simulink model "canudas_goal2"  (R2012b)
settings: Solver=FixedStepDiscrete  StartTime=0.0  StopTime=Inf  FixedStep=0.033  RelTol=1e-3
values from neighbouring files (symbols this model uses):
  eps1 = 0.005    [param.m]
  eps2 = 1*2*pi/360    (= 0.0174532925199)    [param.m]
  k1 = 1.35/4    (= 0.3375)    [param.m]
  k2 = 4.6/4    (= 1.15)    [param.m]
  max_phi = 48000*6.9440e-06/r    (= 16.2591219512)    [param.m]
  max_v = r * max_phi    (= 0.333312)    [param.m]
  max_w = max_phi*2*r/l    (= 7.54014251781)    [param.m]
  thetar = pi    (= 3.14159265359)    [param.m]
  xr = 0    [param.m]
  yr = 0    [param.m]
libraries: simiam x5, simulink x1, simulink_extras x1
settings Model: Creator=jdelacroix  LastModifiedBy=samati
settings DataIOCC: SignalLoggingSaveFormat=ModelDataLogs  SaveOutput=off  SaveTime=off
settings DebuggingCC: MultiTaskDSMMsg=warning  MultiTaskCondExecSysMsg=none  FcnCallInpInsideContextMsg=EnableAllAsWarning  StrictBusMsg=None
settings RTWCC: IncludeERTFirstTime=on
settings CodeAppCC: CustomSymbolStrType=$N$R$M_T  InternalIdentifier=Shortened
settings GRTTargetCC: CodeReplacementLibrary=None  CPPClassGenCompliant=on

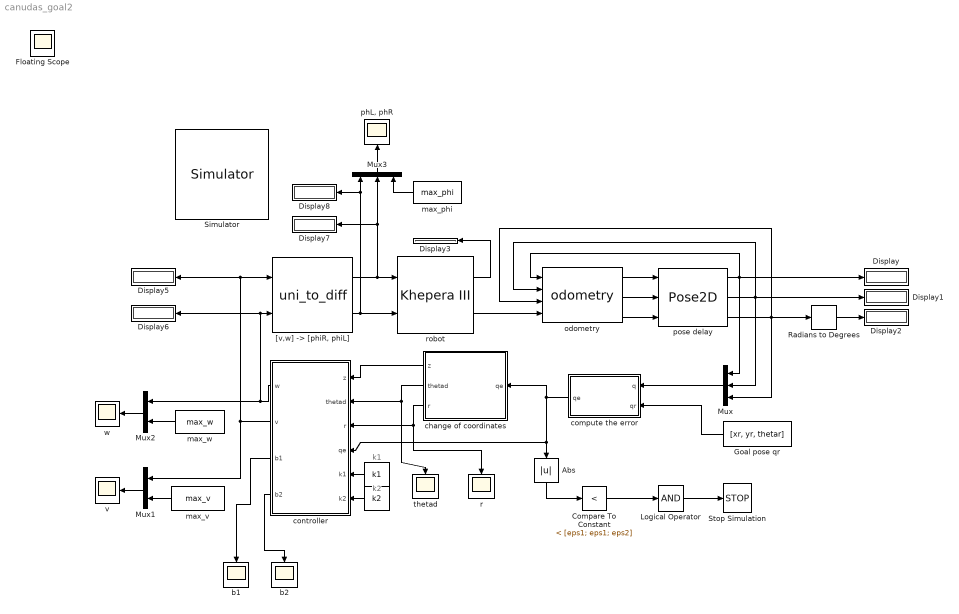
== system canudas_goal2 ==
  note: k2
  note: k1
  " " : Constant  Value=k2
  " " : Constant  Value=k1
  Abs : Abs
  Compare To Constant : simulink/Logic and Bit Operations/Compare To Constant  relop=<  const=[eps1; eps1; eps2]  OutDataTypeStr=boolean
  Display{,1..3,5..8} (8 alike) : Display
  Goal pose qr : Constant  Value=[xr, yr, thetar]
  Logical Operator : Logic  Inputs=1  AllPortsSameDT=off  OutDataTypeStr=boolean
  Mux : Mux  Inputs=3
  Mux1 : Mux  Inputs=2
  Mux2 : Mux  Inputs=2
  Mux3 : Mux  Inputs=3
  Radians to Degrees : simulink_extras/Transformations/Radians to Degrees
  Simulator : simiam/Simulator  Priority=1
  Stop Simulation : Stop
  "[v,w] -> [phiR, phiL]" : simiam/uni_to_diff  wheel_radius=r  wheel_base_length=l
  b1 : Scope
      settings: ShowLegends=on  YMin=-7  YMax=8  SaveName=phiRL4
  b2 : Scope
      settings: ShowLegends=on  YMin=-7  YMax=8  SaveName=phiRL3
  change of coordinates : MATLAB Function  TreatAsAtomicUnit=on
  compute the error : MATLAB Function  TreatAsAtomicUnit=on
  controller : MATLAB Function  TreatAsAtomicUnit=on
  max_phi : Constant  Value=max_phi  OutDataTypeStr=double
  "max_v " : Constant  Value=max_v  OutDataTypeStr=double
  "max_w " : Constant  Value=max_w  OutDataTypeStr=double
  odometry : simiam/odometry  wheel_radius=r  wheel_base_length=l  ticks_per_rev=ticks
  "phL, phR" : Scope
      settings: ShowLegends=on  YMin=-7  YMax=8  SaveName=phiRL
  pose delay : simiam/Pose2D  SystemSampleTime=-1
  r : Scope
      settings: ShowLegends=on  YMin=-7  YMax=8  SaveName=phiRL1
  "robot " : simiam/Khepera III  x_0=xi  y_0=yi  theta_0=thetai  robot_id=1
  thetad : Scope
      settings: ShowLegends=on  TimeRange=10  YMin=-7  YMax=8  SaveName=phiRL2
  v : Scope
      settings: ShowLegends=on  TimeRange=10  YMin=-0.6  YMax=0.55  SaveName=v
  "w " : Scope
      settings: ShowLegends=on  YMin=-0.5  YMax=8  SaveName=w
  Floating Scope : Scope
  wires:
  odometry/2 -> pose delay/2
  odometry/1 -> pose delay/1
  "robot "/2 -> odometry/4
  pose delay/1 -> Mux/1, odometry/1, Display/1
  pose delay/3 -> Mux/3, Radians to Degrees/1, odometry/3
  odometry/3 -> pose delay/3
  "[v,w] -> [phiR, phiL]"/1 -> "robot "/1, Mux3/2, Display7/1
  "[v,w] -> [phiR, phiL]"/2 -> Mux3/1, Display8/1, "robot "/2
  Radians to Degrees/1 -> Display2/1
  "robot "/1 -> Display3/1
  Goal pose qr/1 -> compute the error/2(qr)
  pose delay/2 -> odometry/2, Mux/2, Display1/1
  Mux/1 -> compute the error/1(q)
  controller/1(w) -> Mux2/1, "[v,w] -> [phiR, phiL]"/2, Display6/1
  " "/1 -> controller/5(k1)
  " "/1 -> controller/6(k2)
  controller/2(v) -> "[v,w] -> [phiR, phiL]"/1, Display5/1, Mux1/1
  compute the error/1(qe) -> change of coordinates/1(qe), Abs/1, controller/4(qe)
  Abs/1 -> Compare To Constant/1
  Compare To Constant/1 -> Logical Operator/1
  Logical Operator/1 -> Stop Simulation/1
  "max_v "/1 -> Mux1/2
  Mux1/1 -> v/1
  Mux2/1 -> "w "/1
  "max_w "/1 -> Mux2/2
  Mux3/1 -> "phL, phR"/1
  max_phi/1 -> Mux3/3
  change of coordinates/2(thetad) -> controller/2(thetad), thetad/1
  change of coordinates/3(r) -> r/1, controller/3(r)
  change of coordinates/1(z) -> controller/1(z)
  controller/3(b1) -> b1/1
  controller/4(b2) -> b2/1

== matlab function canudas_goal2/change of coordinates ==
  data: qe input; z output; thetad output; r output
function [z, thetad, r] = aalpha(qe)
% AALPHA Computes the error of the robots pose to the goal pose in other
% coordinates (from (x, y, theta) to (a, alpha)).

% Angle and radius computation
% Check for special case (discontinuity) if xe and ye are zero for thetad
% Check for special case when ye <0 (discontinuity) for a (applied on r)
% Check that thetad and alpha are in ]-pi, pi]
if((abs(qe(1))<eps) && (abs(qe(2))==eps))
    thetad = 0;
else
    thetad = 2*atan2(qe(2),qe(1));
    thetad = limit_angle(thetad);
end

if(abs(qe(2))<eps)
    r = 0;
else
    r = (qe(1)^2 + qe(2)^2)/(2*qe(2));
end

% z computation
a = r * thetad;
alpha = qe(3)-thetad;
alpha = limit_angle(alpha);

z = [a; alpha];

end

== matlab function canudas_goal2/compute the error ==
  data: q input; qe output; qr input
function qe = qe(q, qr)
% QE Compute the error vector qe from the robot to the goal pose.

T = [cos(qr(3)), sin(qr(3)), 0;...
     -sin(qr(3)), cos(qr(3)), 0;...
     0, 0, 1];
 
qe = T*(q-qr);
qe(3) = limit_angle(qe(3));

end

== matlab function canudas_goal2/controller ==
  data: w output; z input; thetad input; r input; v output; qe input; k1 input; k2 input; b1 output; b2 output
function [w, v, b1, b2] = control(z, thetad, r, qe, k1, k2)
% CONTROl Computes the control variables in function of the error z.

b = qe(2)/qe(1);
b1 = cos(qe(3))*(thetad/b - 1) + sin(qe(3))*(thetad*(1 - 1/b^2)/2 + 1/b);
b2 = cos(qe(3))*2*b/((1 + b^2)*qe(1)) - sin(qe(3))*2/((1 + b^2)*qe(1));

v = -k1*b1*z(1);
w = -b2*v-k2*z(2);

end
